simulink model "LAB4_TELEMETRY"  (R2024a)
settings: Solver=FixedStepAuto  StartTime=0.0  StopTime=10  RelTol=1e-8
libraries: instrumentseriallib x2
settings Model: Creator=anton  LastModifiedBy=anton
settings DataIOCC: ExternalInput=data
settings OptimizationCC: ReuseModelBlockBuffer=off
settings DebuggingCC: ParameterPrecisionLossMsg=none
settings RTWCC: GPUComputeCapability=3.5

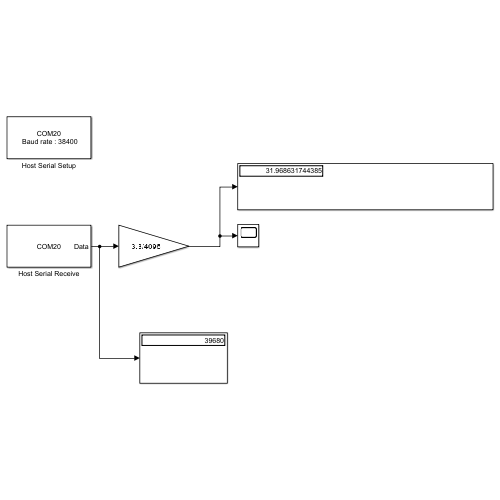
[thumbnail: Simulink's stored preview of the top-level diagram]
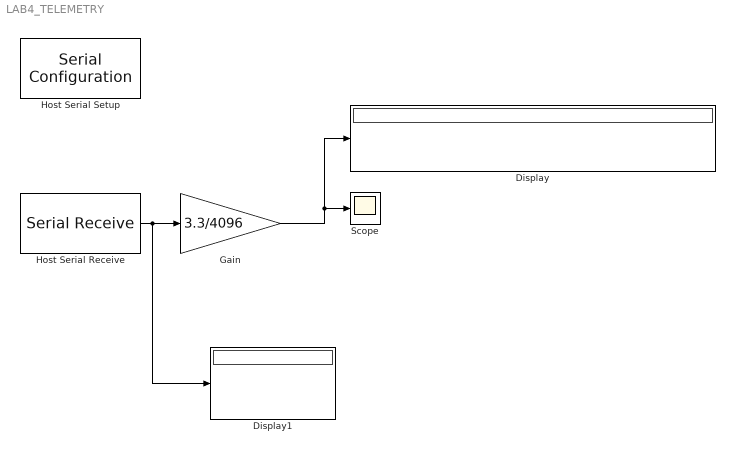
== system LAB4_TELEMETRY ==
  Display : Display
  Display1 : Display
  Gain : Gain  Gain=3.3/4096
  Host Serial Receive : instrumentseriallib/Serial Receive  PortSel=COM20  Port=COM20  ComPort=COM20  DataType=uint32  SaveDataType=uint8  ToggleHeader=on  Header='N'  ToggleDataSize=on  DataSize=1  ToggleTerminator=on  Terminator=Custom terminator  CustomTerminator='E'  InputFormat=Column major  EnableBlockingMode=on  ActionDataUnavailable=Output last received value  ActionWhenDataUnavailable=Output last received value  CustomValue=5  SampleTime=0.01  SimulateUsing=Interpreted execution  BlockInModel=on  aMode=5
      settings: LibrarySourceBlock=mcblib/Protection and Diagnostics/Host Serial Receive
  Host Serial Setup : instrumentseriallib/Serial Configuration  Priority=-99  PortSel=COM20  Port=COM20  ComPort=COM20  BaudRate=38400  DataBits=8  Parity=none  StopBits=1  ByteOrder=little-endian  FlowControl=none  Timeout=1  SimulateUsing=Interpreted execution  BlockInModel=on  aMode=5
      settings: LibrarySourceBlock=mcblib/Protection and Diagnostics/Host Serial Setup
  Scope : Scope
  wires:
  Host Serial Receive/1 -> Display1/1, Gain/1
  Gain/1 -> Display/1, Scope/1
